simulink model "PurePursuitEvasionObstaculos"  (R2021b)
settings: Solver=VariableStepAuto  StartTime=0.0  StopTime=10.0  RelTol=1e-3
settings Model: Creator=ferna  LastModifiedBy=ferna

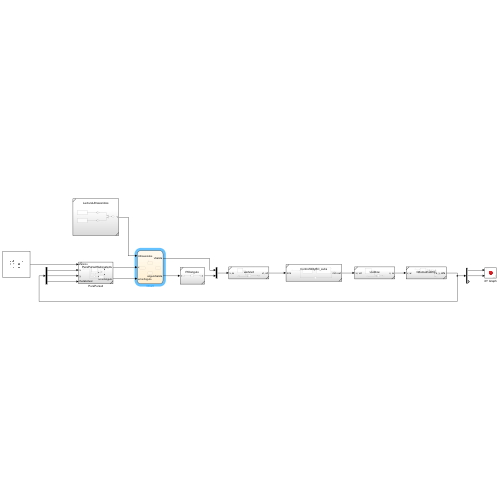
[thumbnail: Simulink's stored preview of the top-level diagram]
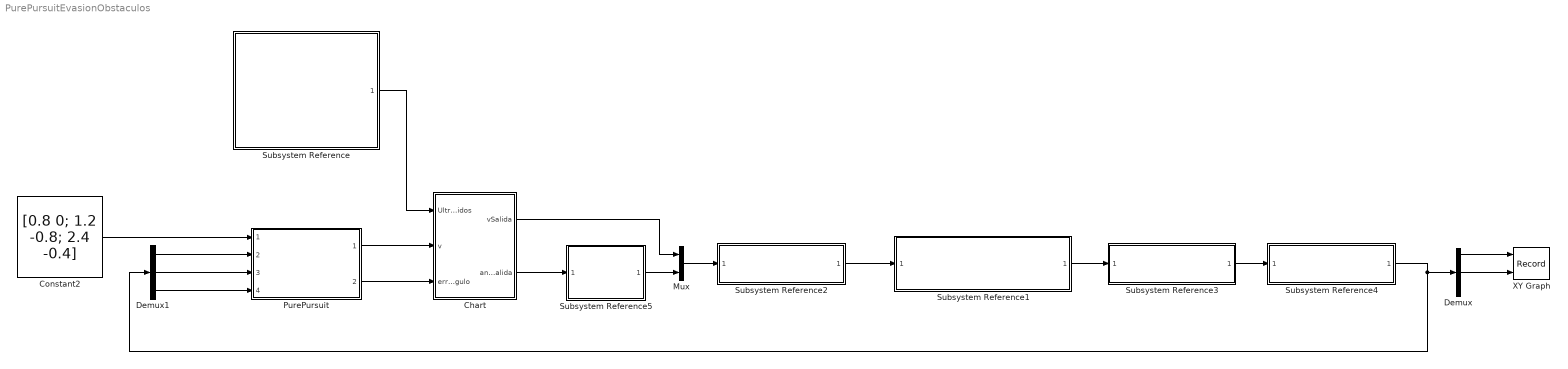
== system PurePursuitEvasionObstaculos ==
  Chart : Stateflow chart  TreatAsAtomicUnit=on
  Constant2 : Constant  Value=[0.8 0; 1.2 -0.8; 2.4 -0.4]  SampleTime=0.01
  Demux : Demux  Outputs=3
  Demux1 : Demux  Outputs=3
  Mux : Mux  Inputs=2
  PurePursuit : Subsystem  ReferencedSubsystem=PurePursuitSubsystem
  Subsystem Reference : Subsystem  ReferencedSubsystem=LecturaUltrasonidos
  Subsystem Reference1 : Subsystem  ReferencedSubsystem=ControlWillyBC_subs
  Subsystem Reference2 : Subsystem  ReferencedSubsystem=vw2vivd
  Subsystem Reference3 : Subsystem  ReferencedSubsystem=vivd2vw
  Subsystem Reference4 : Subsystem  ReferencedSubsystem=OdometriaWilly
  Subsystem Reference5 : Subsystem  ReferencedSubsystem=PIDangulo
  XY Graph : Record  FileSettingsInternal="{\"entries\":[{\"content\":{\"excelSettings\":{\"content\":{},\"type\":\"Streamout.ExcelSettings\"}},\"type\":\"Streamout.FileSettingStorage\",\"uuid\":\"a14bc50a-5f2a-439b-8a9b-59662c4d2e9b\"}],\"packageUris\":[\"http://schema.mathworks.com/mf0/streamout_blocks/R2020a\"],\"version\":\"1.0\"}"  Layout=[1 1]  SignalsInternal="{\"entries\":[{\"content\":{\"signals\":[{\"content\":{\"blockPath\":[\"untitled/XY Graph\"],\"channel\":[],\"dimensions\":[1],\"domain\":\"untitled/XY Graph\",\"lineColor\":\"#a2142f\",\"plots\":[1],\"port\":1,\"sid\":[],\"signalID\":18268,\"signalName\":\"Demux:1\"},\"type\":\"RecordBlkView.Signal\",\"uuid\":\"47203325-4981-4ccd-8073-3120472d8ed1\"},{\"content\":{\"blockPath\":[\"untitled/XY Graph\"],\"channel\":[],\"dimensions\":[1],\"domain\":\"untitled/XY Graph\",\"lineColor\":\"#139fff\",\"plots\":[1],\"port\":2,\"sid\":[],\"signalID\":18271,\"signalName\":\"Demux:2\"},\"type\":\"RecordBlkView.Signal\",\"uuid\":\"fdbc8a80-0acf-40c5-994d-c236eb1578e8\"}]},\"type\":\"RecordBlkView.InputSignals\",\"uuid\":\"c9309e59-ab10-4023-b8e0-f770fe59de6b\"}],\"packageUris\":[\"http://schema.mathworks.com/mf0/streamout_blocks/R2020a\"],\"version\":\"1.0\"}"  VisualizationBindings="{\"xyplotplugin\":{\"info\":[{\"series\":[{\"bindingParametersList\":[{\"parameter\":\"X-Axis\",\"signalID\":18268,\"signalName\":\"Demux:1\"},{\"parameter\":\"Y-Axis\",\"signalID\":18271,\"signalName\":\"Demux:2\"}],\"seriesID\":2480}],\"subplotID\":1}]}}"  CompatibilityTag=XY
  wires:
  Subsystem Reference2/1 -> Subsystem Reference1/1
  Demux/2 -> XY Graph/2
  Subsystem Reference3/1 -> Subsystem Reference4/1
  Subsystem Reference1/1 -> Subsystem Reference3/1
  Mux/1 -> Subsystem Reference2/1
  Subsystem Reference5/1 -> Mux/2
  Subsystem Reference4/1 -> Demux/1, Demux1/1
  Demux/1 -> XY Graph/1
  Constant2/1 -> PurePursuit/1
  Demux1/1 -> PurePursuit/2
  Demux1/2 -> PurePursuit/3
  Demux1/3 -> PurePursuit/4
  PurePursuit/2 -> Chart/3(errorAngulo)
  PurePursuit/1 -> Chart/2(v)
  Subsystem Reference/1 -> Chart/1(Ultrasonidos)
  Chart/1(vSalida) -> Mux/1
  Chart/2(anguloSalida) -> Subsystem Reference5/1

== stateflow chart PurePursuitEvasionObstaculos/Chart ==
  state SinObstaculos
  state ObstaculoIzquierda
  state ObstaculoDerecha
  state ObstaculoAmbos
  (default) -> SinObstaculos
  data: vSalida output; anguloSalida output Enum: ChartModeType; Ultrasonidos input; v input; errorAngulo input
